simulink model "cc"  (R2019b)
settings: Solver=FixedStepAuto  StartTime=0.0  StopTime=5  FixedStep=0.005  RelTol=1e-3  EnableMultiTasking=on
settings Model: Creator=陈晨  LastModifiedBy=陈晨

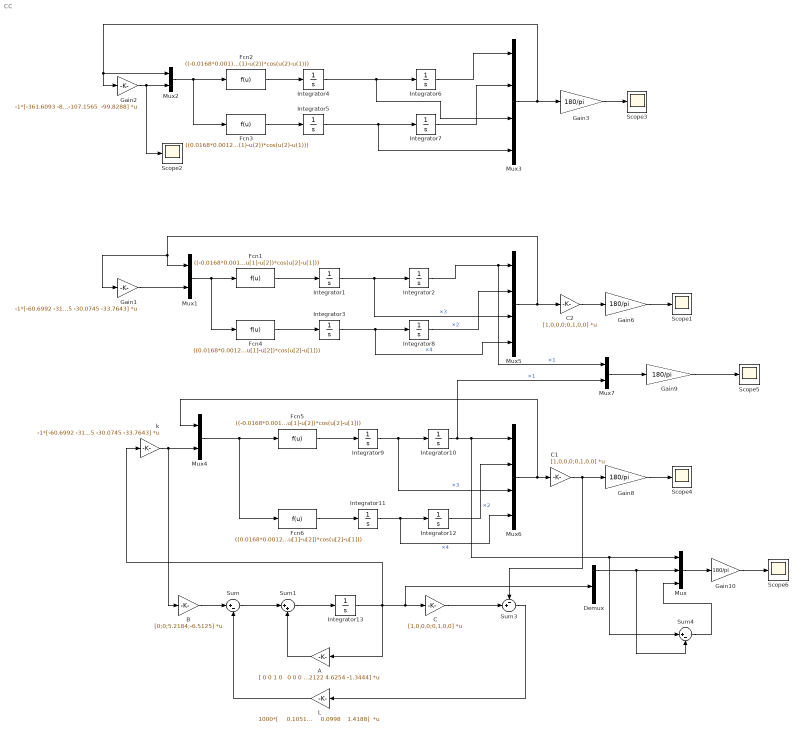
== system cc ==
  A : Gain  Gain=|  Multiplication=Matrix(K*u)
      | [ 0 0 1 0 
      |  0 0 0 1 
      |  65.8751 -16.8751 -3.7062 0.2760 
      |  -82.2122 82.2122 4.6254 -1.3444]
  B : Gain  Gain=[0;0;5.2184;-6.5125]  Multiplication=Matrix(K*u)
  C : Gain  Gain=[1,0,0,0;0,1,0,0]  Multiplication=Matrix(K*u)
  C1 : Gain  Gain=[1,0,0,0;0,1,0,0]  Multiplication=Matrix(K*u)
  C2 : Gain  Gain=[1,0,0,0;0,1,0,0]  Multiplication=Matrix(K*u)
  Demux : Demux
  Fcn1 : Fcn  Expr=((-0.0168*0.001)*u[3]+(0.001*0.0012*cos(u[2]-u[1]))*u[4]+0.0012*0.0012*sin(u[2]-u[1])* cos(u[2]-u[1])*u[3]*u[3]-0.0012*0.001*sin(u[1]-u[2])*u[4]*u[4]+0.2979*0.001*sin(u[1])-0.0612*0.0012*sin(u[2])*cos(u[2]-u[1])+0.0236*0.001*u[5])/(0.0061*0.001-0.0012*0.0012*cos(u[1]-u[2])*cos(u[2]-u[1]))
  Fcn2 : Fcn  Expr=((-0.0168*0.001)*u(3)+(0.001*0.0012*cos(u(2)-u(1)))*u(4)+0.0012*0.0012*sin(u(2)-u(1))* cos(u(2)-u(1))*u(3)*u(3)-0.0012*0.001*sin(u(1)-u(2))*u(4)*u(4)+0.2979*0.001*sin(u(1))-0.0612*0.0012*sin(u(2))*cos(u(2)-u(1))+0.0236*0.001*u(5))/(0.0061*0.001-0.0012*0.0012*cos(u(1)-u(2))*cos(u(2)-u(1)))
  Fcn3 : Fcn  Expr=((0.0168*0.0012*cos(u(1)-u(2)))*u(3)-(0.0061*0.001)*u(4)-0.0061*0.0012*sin(u(2)-u(1))*u(3)*u(3)+0.0012*0.0012*sin(u(1)-u(2))*cos(u(1)-u(2))*u(4)*u(4)-0.2979*0.0012*sin(u(1))*cos(u(1)-u(2))+0.0061*0.0612*sin(u(2))-0.0012*cos(u(1)-u(2))*0.0236*u(5))/(0.0061*0.001-0.0012*0.0012*cos(u(1)-u(2))*cos(u(2)-u(1)))
  Fcn4 : Fcn  Expr=((0.0168*0.0012*cos(u[1]-u[2]))*u[3]-(0.0061*0.001)*u[4]-0.0061*0.0012*sin(u[2]-u[1])*u[3]*u[3]+0.0012*0.0012*sin(u[1]-u[2])*cos(u[1]-u[2])*u[4]*u[4]-0.2979*0.0012*sin(u[1])*cos(u[1]-u[2])+0.0061*0.0612*sin(u[2])-0.0012*cos(u[1]-u[2])*0.0236*u[5])/(0.0061*0.001-0.0012*0.0012*cos(u[1]-u[2])*cos(u[2]-u[1]))
  Fcn5 : Fcn  Expr=((-0.0168*0.001)*u[3]+(0.001*0.0012*cos(u[2]-u[1]))*u[4]+0.0012*0.0012*sin(u[2]-u[1])* cos(u[2]-u[1])*u[3]*u[3]-0.0012*0.001*sin(u[1]-u[2])*u[4]*u[4]+0.2979*0.001*sin(u[1])-0.0612*0.0012*sin(u[2])*cos(u[2]-u[1])+0.0236*0.001*u[5])/(0.0061*0.001-0.0012*0.0012*cos(u[1]-u[2])*cos(u[2]-u[1]))
  Fcn6 : Fcn  Expr=((0.0168*0.0012*cos(u[1]-u[2]))*u[3]-(0.0061*0.001)*u[4]-0.0061*0.0012*sin(u[2]-u[1])*u[3]*u[3]+0.0012*0.0012*sin(u[1]-u[2])*cos(u[1]-u[2])*u[4]*u[4]-0.2979*0.0012*sin(u[1])*cos(u[1]-u[2])+0.0061*0.0612*sin(u[2])-0.0012*cos(u[1]-u[2])*0.0236*u[5])/(0.0061*0.001-0.0012*0.0012*cos(u[1]-u[2])*cos(u[2]-u[1]))
  Gain1 : Gain  Gain=-1*[-60.6992 -316.1745 -30.0745 -33.7643]  Multiplication=Matrix(K*u)
  Gain{3,6,8..10} (5 alike) : Gain  Gain=180/pi
  Gain2 : Gain  Gain="-1*[-361.6093 -856.7554 -107.1565  -99.8288]"  Multiplication=Matrix(K*u)
  Integrator{1,3..5,9,11,13} (7 alike) : Integrator
  Integrator10 : Integrator  InitialCondition=-0.1
  Integrator12 : Integrator  InitialCondition=0.05
  Integrator2 : Integrator  InitialCondition=-0.1
  Integrator6 : Integrator  InitialCondition=-0.1
  Integrator7 : Integrator  InitialCondition=0.05
  Integrator8 : Integrator  InitialCondition=0.05
  L : Gain  Gain=|  Multiplication=Matrix(K*u)
      | 1000*[
      |     0.1051   -0.0216
      |    -0.0108    0.0898
      |     1.8402   -2.1583
      |     0.0998    1.4188]
  Mux : Mux  Inputs=3
  Mux{1..2,4,7} (4 alike) : Mux  Inputs=2
  Mux3 : Mux
  Mux5 : Mux
  Mux6 : Mux
  Scope{1..6} (6 alike) : Scope
  Sum : Sum  Inputs=|+-
  Sum1 : Sum  Inputs=|++
  Sum3 : Sum  Inputs=-+|
  Sum4 : Sum  Inputs=|+-
  k : Gain  Gain=-1*[-60.6992 -316.1745 -30.0745 -33.7643]  Multiplication=Matrix(K*u)
  wires:
  Gain3/1 -> Scope3/1
  Integrator7/1 -> Mux3/2
  Integrator6/1 -> Mux3/1
  Fcn3/1 -> Integrator5/1
  Integrator5/1 -> Mux3/4, Integrator7/1
  Integrator4/1 -> Integrator6/1, Mux3/3
  Mux2/1 -> Fcn3/1, Fcn2/1
  Fcn2/1 -> Integrator4/1
  Gain2/1 -> Scope2/1, Mux2/2
  Mux3/1 -> Mux2/1, Gain2/1, Gain3/1
  Gain1/1 -> Mux1/2
  Mux1/1 -> Fcn4/1, Fcn1/1
  Fcn1/1 -> Integrator1/1
  Integrator1/1 -> Mux5/3, Integrator2/1  "×3"
  Fcn4/1 -> Integrator3/1
  Integrator3/1 -> Integrator8/1, Mux5/4  "×4"
  Mux4/1 -> Fcn6/1, Fcn5/1
  Fcn5/1 -> Integrator9/1
  Integrator9/1 -> Mux6/3, Integrator10/1  "×3"
  Fcn6/1 -> Integrator11/1
  Integrator11/1 -> Mux6/4, Integrator12/1  "×4"
  k/1 -> B/1, Mux4/2
  Integrator2/1 -> Mux7/1, Mux5/1  "×1"
  Integrator8/1 -> Mux5/2  "×2"
  Mux5/1 -> Mux1/1, Gain1/1, C2/1
  C2/1 -> Gain6/1
  Gain6/1 -> Scope1/1
  Integrator10/1 -> Mux6/1, Sum4/1, Mux/1, Mux7/2  "×1"
  Integrator12/1 -> Mux6/2  "×2"
  Mux6/1 -> Mux4/1, C1/1
  C1/1 -> Sum3/1, Gain8/1
  Gain8/1 -> Scope4/1
  Mux7/1 -> Gain9/1
  Gain10/1 -> Scope6/1
  Mux/1 -> Gain10/1
  Demux/1 -> Sum4/2, Mux/2
  Sum4/1 -> Mux/3
  B/1 -> Sum/1
  Sum/1 -> Sum1/1
  Sum1/1 -> Integrator13/1
  A/1 -> Sum1/2
  L/1 -> Sum/2
  Integrator13/1 -> Demux/1, C/1, k/1, A/1
  C/1 -> Sum3/2
  Sum3/1 -> L/1
  Gain9/1 -> Scope5/1
